simulink model "TorqueVect"  (R2022a)
settings: Solver=VariableStepAuto  StartTime=0.0  StopTime=32  RelTol=1e-3
PreLoadFcn:
  | run('Parameters\FSE_Parameters.m')
undefined symbols (not defined in the file): BRegenEnabledButton, canChannel, CyalphaLookUp, efficiency, Fz_curve, Fz_scaling_long, gearR, izz, jw, Kd, kd, Ki, ki, Kp, kp, l_f, l_r, lambda, m, Mz_max, N, N_lat, N_long, P_max, pid_kd_lat, pid_kd_long, pid_ki_lat, pid_ki_long, pid_kp_lat, pid_kp_long, R_max, rw, steerR, T_i_max, TC_Decr_Gas, TC_Derivative, TC_Incr_Gas, TC_On, TC_Relay_Off, TC_Relay_On, tireCornerStiffness, Ts, TV_On, TV_Override, velocity_lookup, velocity_lookup_lat, y_ref, yrr_scaling
libraries: simulink x218, slpidlib x135, CarMaker4SL x101, TractionControlLibrary x13, canmsglib x9, canlib x8, TorqueVectoringLibrary x6, simulink_extras x4, PedalConversionLibrary x3, PowerControlLibrary x1
(part 14 of 26)

== system TorqueVect/CarMaker/IPG Vehicle/PowerTrain/PTControl Example/PTControl_TV_MFE3/Full Control Loop/TC 4 ==
  modified slip ratio reference : Inport
  u_lim : Inport  Port=2
  modified slip ratio measurement : Inport  Port=3
  l_lim : Inport  Port=4
  ResetSignal : Inport  Port=5
  velocity : Inport  Port=6
  Constant : Constant  Value=kp
  Constant1 : Constant  Value=ki
  Constant2 : Constant  Value=kd
  Constant3 : Constant  Value=N
  PID Controller : slpidlib/PID Controller  Controller=PID  Form=Parallel  TimeDomain=Discrete-time  UseExternalTs=off  SampleTime=Ts  IntegratorMethod=Trapezoidal  FilterMethod=Forward Euler  ControllerParametersSource=external  P=kp  I=ki  UseKiTs=on  D=kd  N=100  UseFilter=on  TunerSelectOption=Transfer Function Based (PID Tuner App)  InitialConditionSource=internal  InitialConditionForIntegrator=0  InitialConditionForFilter=0  DifferentiatorICPrevScaledInput=0  ExternalReset=either  TrackingMode=off  Kt=1  LimitOutput=on  SatLimitsSource=external  UpperSaturationLimit=inf  LowerSaturationLimit=-inf  LinearizeAsGain=on  AntiWindupMode=clamping  Kb=1  POutMin=[]  POutMax=[]  IOutMin=[]  IOutMax=[]  DOutMin=[]  DOutMax=[]  NOutMin=[]  NOutMax=[]  SumOutMin=[]  SumOutMax=[]  SaturationOutMin=[]  SaturationOutMax=[]  PParamMin=[]  PParamMax=[]  IParamMin=[]  IParamMax=[]  DParamMin=[]  DParamMax=[]  NParamMin=[]  NParamMax=[]  KbParamMin=[]  KbParamMax=[]  KtParamMin=[]  KtParamMax=[]  KbOutMin=[]  KbOutMax=[]  KtOutMin=[]  KtOutMax=[]  IntegratorOutMin=[]  IntegratorOutMax=[]  FilterOutMin=[]  FilterOutMax=[]  SumI1OutMin=[]  SumI1OutMax=[]  SumI2OutMin=[]  SumI2OutMax=[]  SumI3OutMin=[]  SumI3OutMax=[]  SumI4OutMin=[]  SumI4OutMax=[]  SumDOutMin=[]  SumDOutMax=[]  DifferentiatorOutMin=[]  DifferentiatorOutMax=[]  FilterDiffOutCoefMin=[]  FilterDiffOutCoefMax=[]  ReciprocalOutMin=[]  ReciprocalOutMax=[]  SumDenOutMin=[]  SumDenOutMax=[]  SumNumOutMin=[]  SumNumOutMax=[]  DivideOutMin=[]  DivideOutMax=[]  UdiffTsProdOutMin=[]  UdiffTsProdOutMax=[]  NTsProdOutMin=[]  NTsProdOutMax=[]  UintegralTsProdOutMin=[]  UintegralTsProdOutMax=[]  UngainTsProdOutMin=[]  UngainTsProdOutMax=[]  ClampingZeroOutDataTypeStr=Inherit: Inherit via back propagation  ClampingZeroOutMin=[]  ClampingZeroOutMax=[]  FilterDenConstantOutDataTypeStr=Inherit: Inherit via back propagation  FilterDenConstantOutMin=[]  FilterDenConstantOutMax=[]  PCopyOutDataTypeStr=Inherit: Inherit via back propagation  PCopyOutMin=[]  PCopyOutMax=[]  NCopyOutDataTypeStr=Inherit: Inherit via back propagation  NCopyOutMin=[]  NCopyOutMax=[]  IntegratorContinuousStateAttributes=''  IntegratorStateMustResolveToSignalObject=off  IntegratorRTWStateStorageClass=Auto  FilterContinuousStateAttributes=''  FilterStateMustResolveToSignalObject=off  FilterRTWStateStorageClass=Auto  ParallelPVariant=ExternalParameters  IdealPVariant=Disabled  IVariant=ExternalParameters  DVariant=ExternalParameters  IntegratorVariant=Discrete  SatVariant=External  AWVariant=DiscClampingParallel  PCopyVariant=Disabled  TRVariant=Disabled  FdbkBlocksVariant=Feedback  IdealPFdbkVariant=Passthrough  SatFdbkVariant=Passthrough  DerivativeFilterVariant=ForwardEulerFilter  NVariant=ExternalParameters  NCopyVariant=Disabled  FilterICVariant=InternalICsFilter  IntegratorICVariant=InternalICs  ExternalResetVariant=ExternalReset  TRSumVariant=Passthrough  SumFdbkVariant=Enabled  SumVariant=Sum_PID  TsampFilterVariant=InternalTs  TsampNgainVariant=Passthrough  TsampIntegralVariant=Passthrough  ExternalSaturationOutDataTypeStr=Inherit: Same as second input  aMode=0
  Subsystem : Subsystem
  Sum1 : Sum  Inputs=|+-
  velocity lookup : Constant  Value=velocity_lookup
  Control Effort 1 : Outport
  wires:
  Sum1/1 -> PID Controller/1
  modified slip ratio reference/1 -> Sum1/1
  u_lim/1 -> PID Controller/7
  modified slip ratio measurement/1 -> Sum1/2
  l_lim/1 -> PID Controller/8
  PID Controller/1 -> Control Effort 1/1
  ResetSignal/1 -> PID Controller/6
  velocity/1 -> Subsystem/1(velocity)
  Constant/1 -> Subsystem/2(pid_kp)
  velocity lookup/1 -> Subsystem/3(velocity lookup)
  Subsystem/1(Out1) -> PID Controller/2
  Subsystem/2(Out2) -> PID Controller/3
  Subsystem/3(Out3) -> PID Controller/4
  Constant1/1 -> Subsystem/4(pid_ki)
  Constant2/1 -> Subsystem/5(pid_kd)
  Constant3/1 -> PID Controller/5

== system TorqueVect/CarMaker/IPG Vehicle/PowerTrain/PTControl Example/PTControl_TV_MFE3/New TC/Reference Generator1 ==
  note: For throttle sign and Product:
      | If positive, normal reference
      | If negative (regen), similar reference but negative (negative target slip*times speed), this might need to change to account for regen limits
      | If 0, target zero
  note: Vehicle velocity
  note: Modified slip ratio targets
  x2 : Inport
  Front SR Target : Inport  Port=2
  Rear SR Target : Inport  Port=3
  Constant : Constant
  Product1 : Product
  Product2 : Product
  Switch : Switch  Criteria=u2 > Threshold  Threshold=1  SaturateOnIntegerOverflow=off  InputSameDT=off
  R1 : Outport
  L1 : Outport  Port=2
  R2 : Outport  Port=3
  L2 : Outport  Port=4
  wires:
  Constant/1 -> Switch/3
  x2/1 -> Switch/2, Switch/1
  Switch/1 -> Product1/2, Product2/1
  Rear SR Target/1 -> Product2/2
  Product2/1 -> R2/1, L2/1
  Product1/1 -> R1/1, L1/1
  Front SR Target/1 -> Product1/1

== system TorqueVect/CarMaker/IPG Vehicle/PowerTrain/PTControl Example/PTControl_TV_MFE3/New TC/TC R1 ==
  modified slip ratio reference : Inport
  lim 1 : Inport  Port=2
  modified slip ratio measurement : Inport  Port=3
  P_TC : Inport  Port=4
  D_TC : Inport  Port=5
  enable_tc : Inport  Port=6
  PID Controller : slpidlib/PID Controller  Commented=on  Controller=PD  Form=Parallel  TimeDomain=Discrete-time  UseExternalTs=off  SampleTime=-1  IntegratorMethod=Forward Euler  FilterMethod=Forward Euler  ControllerParametersSource=external  P=125  I=1  UseKiTs=on  D=0  N=100  UseFilter=on  TunerSelectOption=Transfer Function Based (PID Tuner App)  InitialConditionSource=internal  InitialConditionForIntegrator=0  InitialConditionForFilter=0  DifferentiatorICPrevScaledInput=0  ExternalReset=none  TrackingMode=off  Kt=1  LimitOutput=on  SatLimitsSource=external  UpperSaturationLimit=inf  LowerSaturationLimit=-inf  LinearizeAsGain=on  AntiWindupMode=clamping  Kb=1  POutMin=[]  POutMax=[]  IOutMin=[]  IOutMax=[]  DOutMin=[]  DOutMax=[]  NOutMin=[]  NOutMax=[]  SumOutMin=[]  SumOutMax=[]  SaturationOutMin=[]  SaturationOutMax=[]  PParamMin=[]  PParamMax=[]  IParamMin=[]  IParamMax=[]  DParamMin=[]  DParamMax=[]  NParamMin=[]  NParamMax=[]  KbParamMin=[]  KbParamMax=[]  KtParamMin=[]  KtParamMax=[]  KbOutMin=[]  KbOutMax=[]  KtOutMin=[]  KtOutMax=[]  IntegratorOutMin=[]  IntegratorOutMax=[]  FilterOutMin=[]  FilterOutMax=[]  SumI1OutMin=[]  SumI1OutMax=[]  SumI2OutMin=[]  SumI2OutMax=[]  SumI3OutMin=[]  SumI3OutMax=[]  SumI4OutMin=[]  SumI4OutMax=[]  SumDOutMin=[]  SumDOutMax=[]  DifferentiatorOutMin=[]  DifferentiatorOutMax=[]  FilterDiffOutCoefMin=[]  FilterDiffOutCoefMax=[]  ReciprocalOutMin=[]  ReciprocalOutMax=[]  SumDenOutMin=[]  SumDenOutMax=[]  SumNumOutMin=[]  SumNumOutMax=[]  DivideOutMin=[]  DivideOutMax=[]  UdiffTsProdOutMin=[]  UdiffTsProdOutMax=[]  NTsProdOutMin=[]  NTsProdOutMax=[]  UintegralTsProdOutMin=[]  UintegralTsProdOutMax=[]  UngainTsProdOutMin=[]  UngainTsProdOutMax=[]  ClampingZeroOutDataTypeStr=Inherit: Inherit via back propagation  ClampingZeroOutMin=[]  ClampingZeroOutMax=[]  FilterDenConstantOutDataTypeStr=Inherit: Inherit via back propagation  FilterDenConstantOutMin=[]  FilterDenConstantOutMax=[]  PCopyOutDataTypeStr=Inherit: Inherit via back propagation  PCopyOutMin=[]  PCopyOutMax=[]  NCopyOutDataTypeStr=Inherit: Inherit via back propagation  NCopyOutMin=[]  NCopyOutMax=[]  IntegratorContinuousStateAttributes=''  IntegratorStateMustResolveToSignalObject=off  IntegratorRTWStateStorageClass=Auto  FilterContinuousStateAttributes=''  FilterStateMustResolveToSignalObject=off  FilterRTWStateStorageClass=Auto  ParallelPVariant=ExternalParameters  IdealPVariant=Disabled  IVariant=Disabled  DVariant=ExternalParameters  IntegratorVariant=Disabled  SatVariant=External  AWVariant=Disabled  PCopyVariant=Disabled  TRVariant=Disabled  FdbkBlocksVariant=Forward  IdealPFdbkVariant=Disabled  SatFdbkVariant=Disabled  DerivativeFilterVariant=ForwardEulerFilter  NVariant=ExternalParameters  NCopyVariant=Disabled  FilterICVariant=InternalICsFilter  IntegratorICVariant=Disabled  ExternalResetVariant=Disabled  TRSumVariant=Passthrough  SumFdbkVariant=Disabled  SumVariant=Sum_PD  TsampFilterVariant=InternalTs  TsampNgainVariant=Passthrough  TsampIntegralVariant=Disabled_SignalSpec  ExternalSaturationOutDataTypeStr=Inherit: Same as second input  aMode=0
  Sum1 : Sum  Inputs=|-+
  Sum2 : Sum  Commented=on  Inputs=|-+
  traction_controller : Subsystem
  Control Effort 1 : Outport
  wires:
  D_TC/1 -> traction_controller/5(Kd)
  P_TC/1 -> traction_controller/4(Kp)
  Sum1/1 -> traction_controller/2(dslip)
  enable_tc/1 -> traction_controller/3(enable_tc)
  traction_controller/1(delta_torque) -> Control Effort 1/1
  PID Controller/1 -> Sum2/1
  lim 1/1 -> traction_controller/1(max_torque), Sum2/2
  modified slip ratio measurement/1 -> Sum1/2
  modified slip ratio reference/1 -> Sum1/1

== system TorqueVect/CarMaker/IPG Vehicle/PowerTrain/PTControl Example/PTControl_TV_MFE3/New TC/TC R2 ==
  modified slip ratio reference : Inport
  lim 1 : Inport  Port=2
  modified slip ratio measurement : Inport  Port=3
  P_TC : Inport  Port=4
  D_TC : Inport  Port=5
  enable_tc : Inport  Port=6
  PID Controller : slpidlib/PID Controller  Commented=on  Controller=PD  Form=Parallel  TimeDomain=Discrete-time  UseExternalTs=off  SampleTime=-1  IntegratorMethod=Forward Euler  FilterMethod=Forward Euler  ControllerParametersSource=external  P=125  I=1  UseKiTs=on  D=0  N=100  UseFilter=on  TunerSelectOption=Transfer Function Based (PID Tuner App)  InitialConditionSource=internal  InitialConditionForIntegrator=0  InitialConditionForFilter=0  DifferentiatorICPrevScaledInput=0  ExternalReset=none  TrackingMode=off  Kt=1  LimitOutput=on  SatLimitsSource=external  UpperSaturationLimit=inf  LowerSaturationLimit=-inf  LinearizeAsGain=on  AntiWindupMode=clamping  Kb=1  POutMin=[]  POutMax=[]  IOutMin=[]  IOutMax=[]  DOutMin=[]  DOutMax=[]  NOutMin=[]  NOutMax=[]  SumOutMin=[]  SumOutMax=[]  SaturationOutMin=[]  SaturationOutMax=[]  PParamMin=[]  PParamMax=[]  IParamMin=[]  IParamMax=[]  DParamMin=[]  DParamMax=[]  NParamMin=[]  NParamMax=[]  KbParamMin=[]  KbParamMax=[]  KtParamMin=[]  KtParamMax=[]  KbOutMin=[]  KbOutMax=[]  KtOutMin=[]  KtOutMax=[]  IntegratorOutMin=[]  IntegratorOutMax=[]  FilterOutMin=[]  FilterOutMax=[]  SumI1OutMin=[]  SumI1OutMax=[]  SumI2OutMin=[]  SumI2OutMax=[]  SumI3OutMin=[]  SumI3OutMax=[]  SumI4OutMin=[]  SumI4OutMax=[]  SumDOutMin=[]  SumDOutMax=[]  DifferentiatorOutMin=[]  DifferentiatorOutMax=[]  FilterDiffOutCoefMin=[]  FilterDiffOutCoefMax=[]  ReciprocalOutMin=[]  ReciprocalOutMax=[]  SumDenOutMin=[]  SumDenOutMax=[]  SumNumOutMin=[]  SumNumOutMax=[]  DivideOutMin=[]  DivideOutMax=[]  UdiffTsProdOutMin=[]  UdiffTsProdOutMax=[]  NTsProdOutMin=[]  NTsProdOutMax=[]  UintegralTsProdOutMin=[]  UintegralTsProdOutMax=[]  UngainTsProdOutMin=[]  UngainTsProdOutMax=[]  ClampingZeroOutDataTypeStr=Inherit: Inherit via back propagation  ClampingZeroOutMin=[]  ClampingZeroOutMax=[]  FilterDenConstantOutDataTypeStr=Inherit: Inherit via back propagation  FilterDenConstantOutMin=[]  FilterDenConstantOutMax=[]  PCopyOutDataTypeStr=Inherit: Inherit via back propagation  PCopyOutMin=[]  PCopyOutMax=[]  NCopyOutDataTypeStr=Inherit: Inherit via back propagation  NCopyOutMin=[]  NCopyOutMax=[]  IntegratorContinuousStateAttributes=''  IntegratorStateMustResolveToSignalObject=off  IntegratorRTWStateStorageClass=Auto  FilterContinuousStateAttributes=''  FilterStateMustResolveToSignalObject=off  FilterRTWStateStorageClass=Auto  ParallelPVariant=ExternalParameters  IdealPVariant=Disabled  IVariant=Disabled  DVariant=ExternalParameters  IntegratorVariant=Disabled  SatVariant=External  AWVariant=Disabled  PCopyVariant=Disabled  TRVariant=Disabled  FdbkBlocksVariant=Forward  IdealPFdbkVariant=Disabled  SatFdbkVariant=Disabled  DerivativeFilterVariant=ForwardEulerFilter  NVariant=ExternalParameters  NCopyVariant=Disabled  FilterICVariant=InternalICsFilter  IntegratorICVariant=Disabled  ExternalResetVariant=Disabled  TRSumVariant=Passthrough  SumFdbkVariant=Disabled  SumVariant=Sum_PD  TsampFilterVariant=InternalTs  TsampNgainVariant=Passthrough  TsampIntegralVariant=Disabled_SignalSpec  ExternalSaturationOutDataTypeStr=Inherit: Same as second input  aMode=0
  Sum1 : Sum  Inputs=|-+
  Sum2 : Sum  Commented=on  Inputs=|-+
  traction_controller : Subsystem
  Control Effort 1 : Outport
  wires:
  D_TC/1 -> traction_controller/5(Kd)
  P_TC/1 -> traction_controller/4(Kp)
  Sum1/1 -> traction_controller/2(dslip)
  enable_tc/1 -> traction_controller/3(enable_tc)
  traction_controller/1(delta_torque) -> Control Effort 1/1
  PID Controller/1 -> Sum2/1
  lim 1/1 -> traction_controller/1(max_torque), Sum2/2
  modified slip ratio measurement/1 -> Sum1/2
  modified slip ratio reference/1 -> Sum1/1

== system TorqueVect/CarMaker/IPG Vehicle/PowerTrain/PTControl Example/PTControl_TV_MFE3/New TC/TC R3 ==
  modified slip ratio reference : Inport
  lim 1 : Inport  Port=2
  modified slip ratio measurement : Inport  Port=3
  P_TC : Inport  Port=4
  D_TC : Inport  Port=5
  enable_tc : Inport  Port=6
  PID Controller : slpidlib/PID Controller  Commented=on  Controller=PD  Form=Parallel  TimeDomain=Discrete-time  UseExternalTs=off  SampleTime=-1  IntegratorMethod=Forward Euler  FilterMethod=Forward Euler  ControllerParametersSource=external  P=125  I=1  UseKiTs=on  D=0  N=100  UseFilter=on  TunerSelectOption=Transfer Function Based (PID Tuner App)  InitialConditionSource=internal  InitialConditionForIntegrator=0  InitialConditionForFilter=0  DifferentiatorICPrevScaledInput=0  ExternalReset=none  TrackingMode=off  Kt=1  LimitOutput=on  SatLimitsSource=external  UpperSaturationLimit=inf  LowerSaturationLimit=-inf  LinearizeAsGain=on  AntiWindupMode=clamping  Kb=1  POutMin=[]  POutMax=[]  IOutMin=[]  IOutMax=[]  DOutMin=[]  DOutMax=[]  NOutMin=[]  NOutMax=[]  SumOutMin=[]  SumOutMax=[]  SaturationOutMin=[]  SaturationOutMax=[]  PParamMin=[]  PParamMax=[]  IParamMin=[]  IParamMax=[]  DParamMin=[]  DParamMax=[]  NParamMin=[]  NParamMax=[]  KbParamMin=[]  KbParamMax=[]  KtParamMin=[]  KtParamMax=[]  KbOutMin=[]  KbOutMax=[]  KtOutMin=[]  KtOutMax=[]  IntegratorOutMin=[]  IntegratorOutMax=[]  FilterOutMin=[]  FilterOutMax=[]  SumI1OutMin=[]  SumI1OutMax=[]  SumI2OutMin=[]  SumI2OutMax=[]  SumI3OutMin=[]  SumI3OutMax=[]  SumI4OutMin=[]  SumI4OutMax=[]  SumDOutMin=[]  SumDOutMax=[]  DifferentiatorOutMin=[]  DifferentiatorOutMax=[]  FilterDiffOutCoefMin=[]  FilterDiffOutCoefMax=[]  ReciprocalOutMin=[]  ReciprocalOutMax=[]  SumDenOutMin=[]  SumDenOutMax=[]  SumNumOutMin=[]  SumNumOutMax=[]  DivideOutMin=[]  DivideOutMax=[]  UdiffTsProdOutMin=[]  UdiffTsProdOutMax=[]  NTsProdOutMin=[]  NTsProdOutMax=[]  UintegralTsProdOutMin=[]  UintegralTsProdOutMax=[]  UngainTsProdOutMin=[]  UngainTsProdOutMax=[]  ClampingZeroOutDataTypeStr=Inherit: Inherit via back propagation  ClampingZeroOutMin=[]  ClampingZeroOutMax=[]  FilterDenConstantOutDataTypeStr=Inherit: Inherit via back propagation  FilterDenConstantOutMin=[]  FilterDenConstantOutMax=[]  PCopyOutDataTypeStr=Inherit: Inherit via back propagation  PCopyOutMin=[]  PCopyOutMax=[]  NCopyOutDataTypeStr=Inherit: Inherit via back propagation  NCopyOutMin=[]  NCopyOutMax=[]  IntegratorContinuousStateAttributes=''  IntegratorStateMustResolveToSignalObject=off  IntegratorRTWStateStorageClass=Auto  FilterContinuousStateAttributes=''  FilterStateMustResolveToSignalObject=off  FilterRTWStateStorageClass=Auto  ParallelPVariant=ExternalParameters  IdealPVariant=Disabled  IVariant=Disabled  DVariant=ExternalParameters  IntegratorVariant=Disabled  SatVariant=External  AWVariant=Disabled  PCopyVariant=Disabled  TRVariant=Disabled  FdbkBlocksVariant=Forward  IdealPFdbkVariant=Disabled  SatFdbkVariant=Disabled  DerivativeFilterVariant=ForwardEulerFilter  NVariant=ExternalParameters  NCopyVariant=Disabled  FilterICVariant=InternalICsFilter  IntegratorICVariant=Disabled  ExternalResetVariant=Disabled  TRSumVariant=Passthrough  SumFdbkVariant=Disabled  SumVariant=Sum_PD  TsampFilterVariant=InternalTs  TsampNgainVariant=Passthrough  TsampIntegralVariant=Disabled_SignalSpec  ExternalSaturationOutDataTypeStr=Inherit: Same as second input  aMode=0
  Sum1 : Sum  Inputs=|-+
  Sum2 : Sum  Commented=on  Inputs=|-+
  traction_controller : Subsystem
  Control Effort 1 : Outport
  wires:
  D_TC/1 -> traction_controller/5(Kd)
  P_TC/1 -> traction_controller/4(Kp)
  Sum1/1 -> traction_controller/2(dslip)
  enable_tc/1 -> traction_controller/3(enable_tc)
  traction_controller/1(delta_torque) -> Control Effort 1/1
  PID Controller/1 -> Sum2/1
  lim 1/1 -> traction_controller/1(max_torque), Sum2/2
  modified slip ratio measurement/1 -> Sum1/2
  modified slip ratio reference/1 -> Sum1/1

== system TorqueVect/CarMaker/IPG Vehicle/PowerTrain/PTControl Example/PTControl_TV_MFE3/New TC/TC R4 ==
  modified slip ratio reference : Inport
  lim 1 : Inport  Port=2
  modified slip ratio measurement : Inport  Port=3
  P_TC : Inport  Port=4
  D_TC : Inport  Port=5
  enable_tc : Inport  Port=6
  PID Controller : slpidlib/PID Controller  Commented=on  Controller=PD  Form=Parallel  TimeDomain=Discrete-time  UseExternalTs=off  SampleTime=-1  IntegratorMethod=Forward Euler  FilterMethod=Forward Euler  ControllerParametersSource=external  P=125  I=1  UseKiTs=on  D=0  N=100  UseFilter=on  TunerSelectOption=Transfer Function Based (PID Tuner App)  InitialConditionSource=internal  InitialConditionForIntegrator=0  InitialConditionForFilter=0  DifferentiatorICPrevScaledInput=0  ExternalReset=none  TrackingMode=off  Kt=1  LimitOutput=on  SatLimitsSource=external  UpperSaturationLimit=inf  LowerSaturationLimit=-inf  LinearizeAsGain=on  AntiWindupMode=clamping  Kb=1  POutMin=[]  POutMax=[]  IOutMin=[]  IOutMax=[]  DOutMin=[]  DOutMax=[]  NOutMin=[]  NOutMax=[]  SumOutMin=[]  SumOutMax=[]  SaturationOutMin=[]  SaturationOutMax=[]  PParamMin=[]  PParamMax=[]  IParamMin=[]  IParamMax=[]  DParamMin=[]  DParamMax=[]  NParamMin=[]  NParamMax=[]  KbParamMin=[]  KbParamMax=[]  KtParamMin=[]  KtParamMax=[]  KbOutMin=[]  KbOutMax=[]  KtOutMin=[]  KtOutMax=[]  IntegratorOutMin=[]  IntegratorOutMax=[]  FilterOutMin=[]  FilterOutMax=[]  SumI1OutMin=[]  SumI1OutMax=[]  SumI2OutMin=[]  SumI2OutMax=[]  SumI3OutMin=[]  SumI3OutMax=[]  SumI4OutMin=[]  SumI4OutMax=[]  SumDOutMin=[]  SumDOutMax=[]  DifferentiatorOutMin=[]  DifferentiatorOutMax=[]  FilterDiffOutCoefMin=[]  FilterDiffOutCoefMax=[]  ReciprocalOutMin=[]  ReciprocalOutMax=[]  SumDenOutMin=[]  SumDenOutMax=[]  SumNumOutMin=[]  SumNumOutMax=[]  DivideOutMin=[]  DivideOutMax=[]  UdiffTsProdOutMin=[]  UdiffTsProdOutMax=[]  NTsProdOutMin=[]  NTsProdOutMax=[]  UintegralTsProdOutMin=[]  UintegralTsProdOutMax=[]  UngainTsProdOutMin=[]  UngainTsProdOutMax=[]  ClampingZeroOutDataTypeStr=Inherit: Inherit via back propagation  ClampingZeroOutMin=[]  ClampingZeroOutMax=[]  FilterDenConstantOutDataTypeStr=Inherit: Inherit via back propagation  FilterDenConstantOutMin=[]  FilterDenConstantOutMax=[]  PCopyOutDataTypeStr=Inherit: Inherit via back propagation  PCopyOutMin=[]  PCopyOutMax=[]  NCopyOutDataTypeStr=Inherit: Inherit via back propagation  NCopyOutMin=[]  NCopyOutMax=[]  IntegratorContinuousStateAttributes=''  IntegratorStateMustResolveToSignalObject=off  IntegratorRTWStateStorageClass=Auto  FilterContinuousStateAttributes=''  FilterStateMustResolveToSignalObject=off  FilterRTWStateStorageClass=Auto  ParallelPVariant=ExternalParameters  IdealPVariant=Disabled  IVariant=Disabled  DVariant=ExternalParameters  IntegratorVariant=Disabled  SatVariant=External  AWVariant=Disabled  PCopyVariant=Disabled  TRVariant=Disabled  FdbkBlocksVariant=Forward  IdealPFdbkVariant=Disabled  SatFdbkVariant=Disabled  DerivativeFilterVariant=ForwardEulerFilter  NVariant=ExternalParameters  NCopyVariant=Disabled  FilterICVariant=InternalICsFilter  IntegratorICVariant=Disabled  ExternalResetVariant=Disabled  TRSumVariant=Passthrough  SumFdbkVariant=Disabled  SumVariant=Sum_PD  TsampFilterVariant=InternalTs  TsampNgainVariant=Passthrough  TsampIntegralVariant=Disabled_SignalSpec  ExternalSaturationOutDataTypeStr=Inherit: Same as second input  aMode=0
  Sum1 : Sum  Inputs=|-+
  Sum2 : Sum  Commented=on  Inputs=|-+
  traction_controller : Subsystem
  Control Effort 1 : Outport
  wires:
  D_TC/1 -> traction_controller/5(Kd)
  P_TC/1 -> traction_controller/4(Kp)
  Sum1/1 -> traction_controller/2(dslip)
  enable_tc/1 -> traction_controller/3(enable_tc)
  traction_controller/1(delta_torque) -> Control Effort 1/1
  PID Controller/1 -> Sum2/1
  lim 1/1 -> traction_controller/1(max_torque), Sum2/2
  modified slip ratio measurement/1 -> Sum1/2
  modified slip ratio reference/1 -> Sum1/1

== system TorqueVect/CarMaker/IPG Vehicle/PowerTrain/PTControl Example/PTControl_ALL_CTRL_VC_MFE24/New TC/TC R1/traction_controller ==
  max_torque : Inport
  dslip : Inport  Port=2
  enable_tc : Inport  Port=3
  Kp : Inport  Port=4
  Kd : Inport  Port=5
  Add : Sum  Inputs=+-
  Saturation Dynamic : simulink/Discontinuities/Saturation Dynamic  OutMin=[]  OutMax=[]  OutDataTypeStr=Inherit: Same as second input  OutDataType=fixdt(1, 16)  OutScaling=2^-10  DoSatur=off
  min_torque : Constant  Value=0
  traction_controller : Subsystem  TreatAsAtomicUnit=on
  delta_torque : Outport  VectorParamsAs1DForOutWhenUnconnected=off
  wires:
  Kd/1 -> traction_controller/4(Kd)
  enable_tc/1 -> traction_controller/2(enable_tc)
  Kp/1 -> traction_controller/3(Kp)
  traction_controller/1(delta_torque) -> Add/2
  dslip/1 -> traction_controller/1(dslip)
  Saturation Dynamic/1 -> delta_torque/1
  max_torque/1 -> Add/1, Saturation Dynamic/1
  min_torque/1 -> Saturation Dynamic/3
  Add/1 -> Saturation Dynamic/2

== system TorqueVect/CarMaker/IPG Vehicle/PowerTrain/PTControl Example/PTControl_ALL_CTRL_VC_MFE24/New TC/TC R2/traction_controller ==
  max_torque : Inport
  dslip : Inport  Port=2
  enable_tc : Inport  Port=3
  Kp : Inport  Port=4
  Kd : Inport  Port=5
  Add : Sum  Inputs=+-
  Saturation Dynamic : simulink/Discontinuities/Saturation Dynamic  OutMin=[]  OutMax=[]  OutDataTypeStr=Inherit: Same as second input  OutDataType=fixdt(1, 16)  OutScaling=2^-10  DoSatur=off
  min_torque : Constant  Value=0
  traction_controller : Subsystem  TreatAsAtomicUnit=on
  delta_torque : Outport  VectorParamsAs1DForOutWhenUnconnected=off
  wires:
  Kd/1 -> traction_controller/4(Kd)
  enable_tc/1 -> traction_controller/2(enable_tc)
  Kp/1 -> traction_controller/3(Kp)
  traction_controller/1(delta_torque) -> Add/2
  dslip/1 -> traction_controller/1(dslip)
  Saturation Dynamic/1 -> delta_torque/1
  max_torque/1 -> Add/1, Saturation Dynamic/1
  min_torque/1 -> Saturation Dynamic/3
  Add/1 -> Saturation Dynamic/2

== system TorqueVect/CarMaker/IPG Vehicle/PowerTrain/PTControl Example/PTControl_ALL_CTRL_VC_MFE24/New TC/TC R3/traction_controller ==
  max_torque : Inport
  dslip : Inport  Port=2
  enable_tc : Inport  Port=3
  Kp : Inport  Port=4
  Kd : Inport  Port=5
  Add : Sum  Inputs=+-
  Saturation Dynamic : simulink/Discontinuities/Saturation Dynamic  OutMin=[]  OutMax=[]  OutDataTypeStr=Inherit: Same as second input  OutDataType=fixdt(1, 16)  OutScaling=2^-10  DoSatur=off
  min_torque : Constant  Value=0
  traction_controller : Subsystem  TreatAsAtomicUnit=on
  delta_torque : Outport  VectorParamsAs1DForOutWhenUnconnected=off
  wires:
  Kd/1 -> traction_controller/4(Kd)
  enable_tc/1 -> traction_controller/2(enable_tc)
  Kp/1 -> traction_controller/3(Kp)
  traction_controller/1(delta_torque) -> Add/2
  dslip/1 -> traction_controller/1(dslip)
  Saturation Dynamic/1 -> delta_torque/1
  max_torque/1 -> Add/1, Saturation Dynamic/1
  min_torque/1 -> Saturation Dynamic/3
  Add/1 -> Saturation Dynamic/2

== system TorqueVect/CarMaker/IPG Vehicle/PowerTrain/PTControl Example/PTControl_ALL_CTRL_VC_MFE24/New TC/TC R4/traction_controller ==
  max_torque : Inport
  dslip : Inport  Port=2
  enable_tc : Inport  Port=3
  Kp : Inport  Port=4
  Kd : Inport  Port=5
  Add : Sum  Inputs=+-
  Saturation Dynamic : simulink/Discontinuities/Saturation Dynamic  OutMin=[]  OutMax=[]  OutDataTypeStr=Inherit: Same as second input  OutDataType=fixdt(1, 16)  OutScaling=2^-10  DoSatur=off
  min_torque : Constant  Value=0
  traction_controller : Subsystem  TreatAsAtomicUnit=on
  delta_torque : Outport  VectorParamsAs1DForOutWhenUnconnected=off
  wires:
  Kd/1 -> traction_controller/4(Kd)
  enable_tc/1 -> traction_controller/2(enable_tc)
  Kp/1 -> traction_controller/3(Kp)
  traction_controller/1(delta_torque) -> Add/2
  dslip/1 -> traction_controller/1(dslip)
  Saturation Dynamic/1 -> delta_torque/1
  max_torque/1 -> Add/1, Saturation Dynamic/1
  min_torque/1 -> Saturation Dynamic/3
  Add/1 -> Saturation Dynamic/2

== system TorqueVect/CarMaker/IPG Vehicle/PowerTrain/PTControl Example/PTControl_ALL_CTRL_VC_MFE24/Subsystem/PowerControl1/PC PID ==
  PError : Inport
  P_PC : Inport  Port=2
  D_PC : Inport  Port=3
  I_PC : Inport  Port=4
  ResetPID_PC : Inport  Port=5
  MMotorMax : Inport  Port=6
  Constant : Constant  Value=0
  Gain : Gain  Gain=4
  Gain1 : Gain  Gain=0.01
  PID Controller : slpidlib/PID Controller  Controller=PID  Form=Ideal  TimeDomain=Discrete-time  UseExternalTs=off  SampleTime=0.005  IntegratorMethod=Backward Euler  FilterMethod=Forward Euler  ControllerParametersSource=external  P=1  I=1  UseKiTs=on  D=0  N=100  UseFilter=off  TunerSelectOption=Transfer Function Based (PID Tuner App)  InitialConditionSource=internal  InitialConditionForIntegrator=0  InitialConditionForFilter=0  DifferentiatorICPrevScaledInput=0  ExternalReset=rising  TrackingMode=off  Kt=1  LimitOutput=on  SatLimitsSource=external  UpperSaturationLimit=84  LowerSaturationLimit=0  LinearizeAsGain=on  AntiWindupMode=clamping  Kb=2  SaturateOnIntegerOverflow=on  POutMin=[]  POutMax=[]  IOutMin=[]  IOutMax=[]  DOutMin=[]  DOutMax=[]  NOutMin=[]  NOutMax=[]  SumOutMin=[]  SumOutMax=[]  SaturationOutMin=[]  SaturationOutMax=[]  PParamMin=[]  PParamMax=[]  IParamMin=[]  IParamMax=[]  DParamMin=[]  DParamMax=[]  NParamMin=[]  NParamMax=[]  KbParamMin=[]  KbParamMax=[]  KtParamMin=[]  KtParamMax=[]  KbOutMin=[]  KbOutMax=[]  KtOutMin=[]  KtOutMax=[]  IntegratorOutMin=[]  IntegratorOutMax=[]  FilterOutMin=[]  FilterOutMax=[]  SumI1OutMin=[]  SumI1OutMax=[]  SumI2OutMin=[]  SumI2OutMax=[]  SumI3OutMin=[]  SumI3OutMax=[]  SumI4OutMin=[]  SumI4OutMax=[]  SumDOutMin=[]  SumDOutMax=[]  DifferentiatorOutMin=[]  DifferentiatorOutMax=[]  FilterDiffOutCoefMin=[]  FilterDiffOutCoefMax=[]  ReciprocalOutMin=[]  ReciprocalOutMax=[]  SumDenOutMin=[]  SumDenOutMax=[]  SumNumOutMin=[]  SumNumOutMax=[]  DivideOutMin=[]  DivideOutMax=[]  UdiffTsProdOutMin=[]  UdiffTsProdOutMax=[]  NTsProdOutMin=[]  NTsProdOutMax=[]  UintegralTsProdOutMin=[]  UintegralTsProdOutMax=[]  UngainTsProdOutMin=[]  UngainTsProdOutMax=[]  ClampingZeroOutDataTypeStr=Inherit: Inherit via back propagation  ClampingZeroOutMin=[]  ClampingZeroOutMax=[]  FilterDenConstantOutDataTypeStr=Inherit: Inherit via back propagation  FilterDenConstantOutMin=[]  FilterDenConstantOutMax=[]  PCopyOutDataTypeStr=Inherit: Inherit via back propagation  PCopyOutMin=[]  PCopyOutMax=[]  NCopyOutDataTypeStr=Inherit: Inherit via back propagation  NCopyOutMin=[]  NCopyOutMax=[]  IntegratorContinuousStateAttributes=''  IntegratorStateMustResolveToSignalObject=off  IntegratorRTWStateStorageClass=Auto  FilterContinuousStateAttributes=''  FilterStateMustResolveToSignalObject=off  FilterRTWStateStorageClass=Auto  ParallelPVariant=Passthrough  IdealPVariant=ExternalParameters  IVariant=ExternalParameters  DVariant=ExternalParameters  IntegratorVariant=Discrete  SatVariant=External  AWVariant=DiscClampingIdeal  PCopyVariant=ExternalParamsIdeal  TRVariant=Disabled  FdbkBlocksVariant=Feedback  IdealPFdbkVariant=ExternalParameters  SatFdbkVariant=Passthrough  DerivativeFilterVariant=Differentiator  NVariant=Passthrough  NCopyVariant=Disabled_SignalSpec  FilterICVariant=InternalICsDifferentiator  IntegratorICVariant=InternalICs  ExternalResetVariant=ExternalReset  TRSumVariant=Passthrough  SumFdbkVariant=Enabled  SumVariant=Sum_PID  TsampFilterVariant=InternalTs  TsampNgainVariant=Passthrough  TsampIntegralVariant=Passthrough  ExternalSaturationOutDataTypeStr=Inherit: Same as second input  aMode=0
  TrqReductionTotal : Outport
  wires:
  D_PC/1 -> PID Controller/4
  P_PC/1 -> PID Controller/2
  I_PC/1 -> PID Controller/3
  ResetPID_PC/1 -> PID Controller/5
  MMotorMax/1 -> Gain/1
  Gain/1 -> PID Controller/6
  Gain1/1 -> PID Controller/1
  PError/1 -> Gain1/1
  Constant/1 -> PID Controller/7
  PID Controller/1 -> TrqReductionTotal/1

== system TorqueVect/CarMaker/IPG Vehicle/PowerTrain/PTControl Example/PTControl_ALL_CTRL_VC_MFE24/Subsystem/PowerControl1/PID1 ==
  PError : Inport
  PRegenError : Inport  Port=2
  P_PC : Inport  Port=3
  D_PC : Inport  Port=4
  I_PC : Inport  Port=5
  ResetPID_PC : Inport  Port=6
  MMotorMax : Inport  Port=7
  BRegenEnabled : Inport  Port=8
  rThrottlePedal : Inport  Port=9
  AND : Logic  IconShape=distinctive  AllPortsSameDT=off  OutDataTypeStr=boolean
  Add : Sum
  Compare To Constant : simulink/Logic and Bit Operations/Compare To Constant  relop=<=  const=0.1  OutDataTypeStr=boolean
  Constant : Constant  Value=0
  Gain : Gain  Gain=4
  Gain1 : Gain  Gain=0.01
  Gain2 : Gain  Gain=-1
  PID Controller : slpidlib/PID Controller  Controller=PID  Form=Ideal  TimeDomain=Discrete-time  UseExternalTs=off  SampleTime=0.005  IntegratorMethod=Backward Euler  FilterMethod=Forward Euler  ControllerParametersSource=external  P=1  I=1  UseKiTs=on  D=0  N=100  UseFilter=off  TunerSelectOption=Transfer Function Based (PID Tuner App)  InitialConditionSource=internal  InitialConditionForIntegrator=0  InitialConditionForFilter=0  DifferentiatorICPrevScaledInput=0  ExternalReset=rising  TrackingMode=off  Kt=1  LimitOutput=on  SatLimitsSource=external  UpperSaturationLimit=84  LowerSaturationLimit=0  LinearizeAsGain=on  AntiWindupMode=clamping  Kb=2  SaturateOnIntegerOverflow=on  POutMin=[]  POutMax=[]  IOutMin=[]  IOutMax=[]  DOutMin=[]  DOutMax=[]  NOutMin=[]  NOutMax=[]  SumOutMin=[]  SumOutMax=[]  SaturationOutMin=[]  SaturationOutMax=[]  PParamMin=[]  PParamMax=[]  IParamMin=[]  IParamMax=[]  DParamMin=[]  DParamMax=[]  NParamMin=[]  NParamMax=[]  KbParamMin=[]  KbParamMax=[]  KtParamMin=[]  KtParamMax=[]  KbOutMin=[]  KbOutMax=[]  KtOutMin=[]  KtOutMax=[]  IntegratorOutMin=[]  IntegratorOutMax=[]  FilterOutMin=[]  FilterOutMax=[]  SumI1OutMin=[]  SumI1OutMax=[]  SumI2OutMin=[]  SumI2OutMax=[]  SumI3OutMin=[]  SumI3OutMax=[]  SumI4OutMin=[]  SumI4OutMax=[]  SumDOutMin=[]  SumDOutMax=[]  DifferentiatorOutMin=[]  DifferentiatorOutMax=[]  FilterDiffOutCoefMin=[]  FilterDiffOutCoefMax=[]  ReciprocalOutMin=[]  ReciprocalOutMax=[]  SumDenOutMin=[]  SumDenOutMax=[]  SumNumOutMin=[]  SumNumOutMax=[]  DivideOutMin=[]  DivideOutMax=[]  UdiffTsProdOutMin=[]  UdiffTsProdOutMax=[]  NTsProdOutMin=[]  NTsProdOutMax=[]  UintegralTsProdOutMin=[]  UintegralTsProdOutMax=[]  UngainTsProdOutMin=[]  UngainTsProdOutMax=[]  ClampingZeroOutDataTypeStr=Inherit: Inherit via back propagation  ClampingZeroOutMin=[]  ClampingZeroOutMax=[]  FilterDenConstantOutDataTypeStr=Inherit: Inherit via back propagation  FilterDenConstantOutMin=[]  FilterDenConstantOutMax=[]  PCopyOutDataTypeStr=Inherit: Inherit via back propagation  PCopyOutMin=[]  PCopyOutMax=[]  NCopyOutDataTypeStr=Inherit: Inherit via back propagation  NCopyOutMin=[]  NCopyOutMax=[]  IntegratorContinuousStateAttributes=''  IntegratorStateMustResolveToSignalObject=off  IntegratorRTWStateStorageClass=Auto  FilterContinuousStateAttributes=''  FilterStateMustResolveToSignalObject=off  FilterRTWStateStorageClass=Auto  ParallelPVariant=Passthrough  IdealPVariant=ExternalParameters  IVariant=ExternalParameters  DVariant=ExternalParameters  IntegratorVariant=Discrete  SatVariant=External  AWVariant=DiscClampingIdeal  PCopyVariant=ExternalParamsIdeal  TRVariant=Disabled  FdbkBlocksVariant=Feedback  IdealPFdbkVariant=ExternalParameters  SatFdbkVariant=Passthrough  DerivativeFilterVariant=Differentiator  NVariant=Passthrough  NCopyVariant=Disabled_SignalSpec  FilterICVariant=InternalICsDifferentiator  IntegratorICVariant=InternalICs  ExternalResetVariant=ExternalReset  TRSumVariant=Passthrough  SumFdbkVariant=Enabled  SumVariant=Sum_PID  TsampFilterVariant=InternalTs  TsampNgainVariant=Passthrough  TsampIntegralVariant=Passthrough  ExternalSaturationOutDataTypeStr=Inherit: Same as second input  aMode=0
  Switch : Switch  Criteria=u2 > Threshold  SaturateOnIntegerOverflow=off  InputSameDT=off
  TrqReductionTotal : Outport
  wires:
  ? -> TrqReductionTotal/1  "control input delta_P"
  D_PC/1 -> ?
  P_PC/1 -> ?
  I_PC/1 -> ?
  ResetPID_PC/1 -> ?
  MMotorMax/1 -> Gain/1
  Gain/1 -> Gain2/1
  Gain1/1 -> ?
  Add/1 -> Gain1/1
  PError/1 -> Add/1
  PRegenError/1 -> Add/2
  rThrottlePedal/1 -> ?
  BRegenEnabled/1 -> AND/1
  ? -> AND/2
  AND/1 -> Switch/2
  Switch/1 -> ?
  Constant/1 -> Switch/3
  Gain2/1 -> Switch/1

== system TorqueVect/CarMaker/IPG Vehicle/PowerTrain/PTControl Example/PTControl_ALL_CTRL_VC_MFE24/Subsystem/PowerControl1/PowerError ==
  PPositiveTotal : Inport  Unit=W  PortDimensions=1
      settings: AttributesFormatString=%<Unit>
  FF_PC : Inport  Port=2
  PLimit : Inport  Port=3  OutMin=0  OutMax=80000  Unit=W  PortDimensions=1
      settings: AttributesFormatString=[%<OutMin>, %<OutMax>] %<Unit>
  Product5 : Product
  Saturation2 : Saturate  UpperLimit=250000  LowerLimit=0
      settings: AttributesFormatString=[%<LowerLimit>, %<UpperLimit>] W
  Subtract2 : Sum  Inputs=+-
  PError : Outport  Unit=W  PortDimensions=1
      settings: AttributesFormatString=%<Unit>
  wires:
  FF_PC/1 -> Product5/2
  Subtract2/1 -> Saturation2/1
  PLimit/1 -> Subtract2/2
  PPositiveTotal/1 -> Product5/1
  Saturation2/1 -> PError/1  "power error"
  Product5/1 -> Subtract2/1

== system TorqueVect/CarMaker/IPG Vehicle/PowerTrain/PTControl Example/PTControl_ALL_CTRL_VC_MFE24/Subsystem/PowerControl1/RC PID ==
  PRegenError : Inport
  P_RC : Inport  Port=2
  D_RC : Inport  Port=3
  I_RC : Inport  Port=4
  ResetPID_RC : Inport  Port=5
  MRegenMotorMax : Inport  Port=6
  Constant : Constant  Value=0
  Gain : Gain  Gain=-4
  Gain1 : Gain  Gain=-0.01
  PID Controller : slpidlib/PID Controller  Controller=PID  Form=Ideal  TimeDomain=Discrete-time  UseExternalTs=off  SampleTime=0.005  IntegratorMethod=Backward Euler  FilterMethod=Forward Euler  ControllerParametersSource=external  P=1  I=1  UseKiTs=on  D=0  N=100  UseFilter=off  TunerSelectOption=Transfer Function Based (PID Tuner App)  InitialConditionSource=internal  InitialConditionForIntegrator=0  InitialConditionForFilter=0  DifferentiatorICPrevScaledInput=0  ExternalReset=level  TrackingMode=off  Kt=1  LimitOutput=on  SatLimitsSource=external  UpperSaturationLimit=84  LowerSaturationLimit=0  LinearizeAsGain=on  AntiWindupMode=clamping  Kb=2  SaturateOnIntegerOverflow=on  POutMin=[]  POutMax=[]  IOutMin=[]  IOutMax=[]  DOutMin=[]  DOutMax=[]  NOutMin=[]  NOutMax=[]  SumOutMin=[]  SumOutMax=[]  SaturationOutMin=[]  SaturationOutMax=[]  PParamMin=[]  PParamMax=[]  IParamMin=[]  IParamMax=[]  DParamMin=[]  DParamMax=[]  NParamMin=[]  NParamMax=[]  KbParamMin=[]  KbParamMax=[]  KtParamMin=[]  KtParamMax=[]  KbOutMin=[]  KbOutMax=[]  KtOutMin=[]  KtOutMax=[]  IntegratorOutMin=[]  IntegratorOutMax=[]  FilterOutMin=[]  FilterOutMax=[]  SumI1OutMin=[]  SumI1OutMax=[]  SumI2OutMin=[]  SumI2OutMax=[]  SumI3OutMin=[]  SumI3OutMax=[]  SumI4OutMin=[]  SumI4OutMax=[]  SumDOutMin=[]  SumDOutMax=[]  DifferentiatorOutMin=[]  DifferentiatorOutMax=[]  FilterDiffOutCoefMin=[]  FilterDiffOutCoefMax=[]  ReciprocalOutMin=[]  ReciprocalOutMax=[]  SumDenOutMin=[]  SumDenOutMax=[]  SumNumOutMin=[]  SumNumOutMax=[]  DivideOutMin=[]  DivideOutMax=[]  UdiffTsProdOutMin=[]  UdiffTsProdOutMax=[]  NTsProdOutMin=[]  NTsProdOutMax=[]  UintegralTsProdOutMin=[]  UintegralTsProdOutMax=[]  UngainTsProdOutMin=[]  UngainTsProdOutMax=[]  ClampingZeroOutDataTypeStr=Inherit: Inherit via back propagation  ClampingZeroOutMin=[]  ClampingZeroOutMax=[]  FilterDenConstantOutDataTypeStr=Inherit: Inherit via back propagation  FilterDenConstantOutMin=[]  FilterDenConstantOutMax=[]  PCopyOutDataTypeStr=Inherit: Inherit via back propagation  PCopyOutMin=[]  PCopyOutMax=[]  NCopyOutDataTypeStr=Inherit: Inherit via back propagation  NCopyOutMin=[]  NCopyOutMax=[]  IntegratorContinuousStateAttributes=''  IntegratorStateMustResolveToSignalObject=off  IntegratorRTWStateStorageClass=Auto  FilterContinuousStateAttributes=''  FilterStateMustResolveToSignalObject=off  FilterRTWStateStorageClass=Auto  ParallelPVariant=Passthrough  IdealPVariant=ExternalParameters  IVariant=ExternalParameters  DVariant=ExternalParameters  IntegratorVariant=Discrete  SatVariant=External  AWVariant=DiscClampingIdeal  PCopyVariant=ExternalParamsIdeal  TRVariant=Disabled  FdbkBlocksVariant=Feedback  IdealPFdbkVariant=ExternalParameters  SatFdbkVariant=Passthrough  DerivativeFilterVariant=Differentiator  NVariant=Passthrough  NCopyVariant=Disabled_SignalSpec  FilterICVariant=InternalICsDifferentiator  IntegratorICVariant=InternalICs  ExternalResetVariant=ExternalReset  TRSumVariant=Passthrough  SumFdbkVariant=Enabled  SumVariant=Sum_PID  TsampFilterVariant=InternalTs  TsampNgainVariant=Passthrough  TsampIntegralVariant=Passthrough  ExternalSaturationOutDataTypeStr=Inherit: Same as second input  aMode=0
  RegenTrqReductionTotal : Outport
  wires:
  D_RC/1 -> PID Controller/4
  P_RC/1 -> PID Controller/2
  I_RC/1 -> PID Controller/3
  ResetPID_RC/1 -> PID Controller/5
  Gain1/1 -> PID Controller/1
  PRegenError/1 -> Gain1/1
  MRegenMotorMax/1 -> Gain/1
  Constant/1 -> PID Controller/6
  Gain/1 -> PID Controller/7
  PID Controller/1 -> RegenTrqReductionTotal/1

== system TorqueVect/CarMaker/IPG Vehicle/PowerTrain/PTControl Example/PTControl_ALL_CTRL_VC_MFE24/Subsystem/PowerControl1/RegenError ==
  PTotal : Inport  Unit=W  PortDimensions=1
      settings: AttributesFormatString=%<Unit>
  FF_RC : Inport  Port=2
  PRegenLimit : Inport  Port=3  OutMin=0  OutMax=80000  Unit=W  PortDimensions=1
      settings: AttributesFormatString=[%<OutMin>, %<OutMax>] %<Unit>
  rThrottle : Inport  Port=4
  BRegenEnable : Inport  Port=5
  Product : Product
  Product1 : Product
  Product6 : Product
  Saturation : Saturate  UpperLimit=0  LowerLimit=-250000
  Saturation7 : Saturate  UpperLimit=0  LowerLimit=-250000
      settings: AttributesFormatString=[%<LowerLimit>, %<UpperLimit>] W
  Subtract1 : Sum  Inputs=+-
  PRegenError : Outport  Unit=W  PortDimensions=1
      settings: AttributesFormatString=%<Unit>
  wires:
  Saturation/1 -> Subtract1/2
  PRegenLimit/1 -> Product/2
  rThrottle/1 -> Product/1
  Product/1 -> Saturation/1
  Subtract1/1 -> Saturation7/1
  PTotal/1 -> Product6/1
  Product6/1 -> Subtract1/1
  FF_RC/1 -> Product6/2
  Product1/1 -> PRegenError/1
  Saturation7/1 -> Product1/1  "regen error"
  BRegenEnable/1 -> Product1/2

== system TorqueVect/CarMaker/IPG Vehicle/PowerTrain/PTControl Example/PTControl_ALL_CTRL_VC_MFE24/Subsystem/PowerControl1/ResetPID_PC ==
  note: Resets when the pedal is below pos torque demand and there is still a reduction by the PID
  note: Resets when the pedal is in the idle zone [8-11%]
  rThrottlePedal : Inport
  PReductionTotal : Inport  Port=2
  AND : Logic  IconShape=distinctive  AllPortsSameDT=off  OutDataTypeStr=boolean
  AND1 : Logic  Inputs=3  IconShape=distinctive  AllPortsSameDT=off  OutDataTypeStr=boolean
  Compare To Constant1 : simulink/Logic and Bit Operations/Compare To Constant  relop=<=  const=0.1  OutDataTypeStr=boolean
  Compare To Constant2 : simulink/Logic and Bit Operations/Compare To Constant  relop=<=  const=0.11  OutDataTypeStr=boolean
  Compare To Constant3 : simulink/Logic and Bit Operations/Compare To Constant  relop=>=  const=0.08  OutDataTypeStr=boolean
  Compare To Constant4 : simulink/Logic and Bit Operations/Compare To Constant  relop=>  const=0  OutDataTypeStr=boolean
  Detect Fall Negative1 : simulink/Logic and Bit Operations/Detect Fall Negative  vinit=0  OutDataTypeStr=boolean
      settings: SourceProductBaseCode=SL
  Discrete Derivative1 : simulink/Discrete/Discrete Derivative  gainval=1.0  ICPrevScaledInput=0.0  OutMin=[]  OutMax=[]  OutDataType=fixdt(1, 16)  OutScaling=2^-10  DoSatur=off
  OR : Logic  Operator=OR  IconShape=distinctive  AllPortsSameDT=off  OutDataTypeStr=boolean
  ResetPID_PC : Outport
  wires:
  rThrottlePedal/1 -> Compare To Constant2/1, Discrete Derivative1/1, Compare To Constant3/1, Compare To Constant1/1
  OR/1 -> ResetPID_PC/1
  PReductionTotal/1 -> Compare To Constant4/1
  AND1/1 -> OR/1
  AND/1 -> OR/2
  Compare To Constant2/1 -> AND1/3
  Discrete Derivative1/1 -> Detect Fall Negative1/1
  Detect Fall Negative1/1 -> AND1/2
  Compare To Constant3/1 -> AND/1
  Compare To Constant1/1 -> AND/2

== system TorqueVect/CarMaker/IPG Vehicle/PowerTrain/PTControl Example/PTControl_ALL_CTRL_VC_MFE24/Subsystem/PowerControl1/ResetPID_RC ==
  note: Resets when the pedal is above regen torque demand and there is still a reaction by the PID
  note: Resets when regen becomes disabled
  note: Resets when the pedal is in the idle zone [8-11%]
  rThrottlePedal1 : Inport
  RegenTrqReductionTotal1 : Inport  Port=2
  BRegenEnabled1 : Inport  Port=3
  Current : Inport  Port=4
  AND2 : Logic  IconShape=distinctive  AllPortsSameDT=off  OutDataTypeStr=boolean
  AND3 : Logic  Inputs=3  IconShape=distinctive  AllPortsSameDT=off  OutDataTypeStr=boolean
  Compare To Constant10 : simulink/Logic and Bit Operations/Compare To Constant  relop=<  const=0  OutDataTypeStr=boolean
  Compare To Constant11 : simulink/Logic and Bit Operations/Compare To Constant  relop=>=  const=0  OutDataTypeStr=boolean
  Compare To Constant6 : simulink/Logic and Bit Operations/Compare To Constant  relop===  const=0  OutDataTypeStr=boolean
  Compare To Constant7 : simulink/Logic and Bit Operations/Compare To Constant  relop=>=  const=0.07  OutDataTypeStr=boolean
  Compare To Constant8 : simulink/Logic and Bit Operations/Compare To Constant  relop=<=  const=0.1  OutDataTypeStr=boolean
  Compare To Constant9 : simulink/Logic and Bit Operations/Compare To Constant  relop=>=  const=0.07  OutDataTypeStr=boolean
  Detect Fall Negative1 : simulink/Logic and Bit Operations/Detect Fall Negative  vinit=0  OutDataTypeStr=boolean
      settings: SourceProductBaseCode=SL
  Detect Rise Positive1 : simulink/Logic and Bit Operations/Detect Rise Positive  vinit=0  OutDataTypeStr=boolean
  Discrete Derivative2 : simulink/Discrete/Discrete Derivative  gainval=1.0  ICPrevScaledInput=0.0  OutMin=[]  OutMax=[]  OutDataType=fixdt(1, 16)  OutScaling=2^-10  DoSatur=off
  OR2 : Logic  Operator=OR  Inputs=4  IconShape=distinctive  AllPortsSameDT=off  OutDataTypeStr=boolean
  OR3 : Logic  Operator=OR  IconShape=distinctive  AllPortsSameDT=off  OutDataTypeStr=boolean
  ResetPID_RC1 : Outport
  wires:
  AND3/1 -> OR2/2
  BRegenEnabled1/1 -> Compare To Constant6/1, Detect Fall Negative1/1
  Compare To Constant7/1 -> AND2/1
  Compare To Constant9/1 -> AND3/3
  Detect Fall Negative1/1 -> OR3/2
  Compare To Constant6/1 -> OR3/1
  Current/1 -> Compare To Constant11/1
  Compare To Constant11/1 -> OR2/4
  Detect Rise Positive1/1 -> AND3/2  "accel_pedal_rising_or"
  OR2/1 -> ResetPID_RC1/1
  OR3/1 -> OR2/1
  AND2/1 -> OR2/3
  Compare To Constant8/1 -> AND3/1
  Discrete Derivative2/1 -> Detect Rise Positive1/1
  RegenTrqReductionTotal1/1 -> Compare To Constant10/1
  Compare To Constant10/1 -> AND2/2
  rThrottlePedal1/1 -> Compare To Constant7/1, Compare To Constant9/1, Compare To Constant8/1, Discrete Derivative2/1

== system TorqueVect/CarMaker/IPG Vehicle/PowerTrain/PTControl Example/PTControl_ALL_CTRL_VC_MFE24/Subsystem/PowerControl1/Subsystem ==
  TrqReductionTotal : Inport
  rSplitF : Inport  Port=2
  Constant : Constant
  Product : Product
  Sum : Sum  Inputs=|+-
  Sum1 : Sum  Inputs=|-+
  TrqReductionR : Outport
  TrqReductionF : Outport  Port=2
  wires:
  TrqReductionTotal/1 -> Product/1, Sum/1
  Product/1 -> TrqReductionF/1, Sum/2
  Sum/1 -> TrqReductionR/1
  rSplitF/1 -> Sum1/1
  Constant/1 -> Sum1/2
  Sum1/1 -> Product/2

== system TorqueVect/CarMaker/IPG Vehicle/PowerTrain/PTControl Example/PTControl_ALL_CTRL_VC_MFE24/Subsystem/PowerControl1/TotalPower ==
  PMeasured : Inport  OutMin=-250000  OutMax=250000  Unit=W  PortDimensions=1
      settings: AttributesFormatString=[%<OutMin>, %<OutMax>] %<Unit>
  Saturation5 : Saturate  UpperLimit=250000  LowerLimit=0
  PPositiveTotal : Outport  OutMin=0  OutMax=250000  Unit=W  PortDimensions=1
      settings: AttributesFormatString=[%<OutMin>, %<OutMax>] %<Unit>
  PTotal : Outport  Port=2
  wires:
  PMeasured/1 -> PTotal/1, Saturation5/1
  Saturation5/1 -> PPositiveTotal/1

== system TorqueVect/CarMaker/IPG Vehicle/PowerTrain/PTControl Example/PTControl_ALL_CTRL_VC_MFE24/Subsystem/PowerControl2/PC PID ==
  PError : Inport
  P_PC : Inport  Port=2
  D_PC : Inport  Port=3
  I_PC : Inport  Port=4
  ResetPID_PC : Inport  Port=5
  MMotorMax : Inport  Port=6
  Constant : Constant  Value=0
  Gain : Gain  Gain=4
  Gain1 : Gain  Gain=0.01
  PID Controller : slpidlib/PID Controller  Controller=PID  Form=Ideal  TimeDomain=Discrete-time  UseExternalTs=off  SampleTime=0.005  IntegratorMethod=Backward Euler  FilterMethod=Forward Euler  ControllerParametersSource=external  P=1  I=1  UseKiTs=on  D=0  N=100  UseFilter=off  TunerSelectOption=Transfer Function Based (PID Tuner App)  InitialConditionSource=internal  InitialConditionForIntegrator=0  InitialConditionForFilter=0  DifferentiatorICPrevScaledInput=0  ExternalReset=rising  TrackingMode=off  Kt=1  LimitOutput=on  SatLimitsSource=external  UpperSaturationLimit=84  LowerSaturationLimit=0  LinearizeAsGain=on  AntiWindupMode=clamping  Kb=2  SaturateOnIntegerOverflow=on  POutMin=[]  POutMax=[]  IOutMin=[]  IOutMax=[]  DOutMin=[]  DOutMax=[]  NOutMin=[]  NOutMax=[]  SumOutMin=[]  SumOutMax=[]  SaturationOutMin=[]  SaturationOutMax=[]  PParamMin=[]  PParamMax=[]  IParamMin=[]  IParamMax=[]  DParamMin=[]  DParamMax=[]  NParamMin=[]  NParamMax=[]  KbParamMin=[]  KbParamMax=[]  KtParamMin=[]  KtParamMax=[]  KbOutMin=[]  KbOutMax=[]  KtOutMin=[]  KtOutMax=[]  IntegratorOutMin=[]  IntegratorOutMax=[]  FilterOutMin=[]  FilterOutMax=[]  SumI1OutMin=[]  SumI1OutMax=[]  SumI2OutMin=[]  SumI2OutMax=[]  SumI3OutMin=[]  SumI3OutMax=[]  SumI4OutMin=[]  SumI4OutMax=[]  SumDOutMin=[]  SumDOutMax=[]  DifferentiatorOutMin=[]  DifferentiatorOutMax=[]  FilterDiffOutCoefMin=[]  FilterDiffOutCoefMax=[]  ReciprocalOutMin=[]  ReciprocalOutMax=[]  SumDenOutMin=[]  SumDenOutMax=[]  SumNumOutMin=[]  SumNumOutMax=[]  DivideOutMin=[]  DivideOutMax=[]  UdiffTsProdOutMin=[]  UdiffTsProdOutMax=[]  NTsProdOutMin=[]  NTsProdOutMax=[]  UintegralTsProdOutMin=[]  UintegralTsProdOutMax=[]  UngainTsProdOutMin=[]  UngainTsProdOutMax=[]  ClampingZeroOutDataTypeStr=Inherit: Inherit via back propagation  ClampingZeroOutMin=[]  ClampingZeroOutMax=[]  FilterDenConstantOutDataTypeStr=Inherit: Inherit via back propagation  FilterDenConstantOutMin=[]  FilterDenConstantOutMax=[]  PCopyOutDataTypeStr=Inherit: Inherit via back propagation  PCopyOutMin=[]  PCopyOutMax=[]  NCopyOutDataTypeStr=Inherit: Inherit via back propagation  NCopyOutMin=[]  NCopyOutMax=[]  IntegratorContinuousStateAttributes=''  IntegratorStateMustResolveToSignalObject=off  IntegratorRTWStateStorageClass=Auto  FilterContinuousStateAttributes=''  FilterStateMustResolveToSignalObject=off  FilterRTWStateStorageClass=Auto  ParallelPVariant=Passthrough  IdealPVariant=ExternalParameters  IVariant=ExternalParameters  DVariant=ExternalParameters  IntegratorVariant=Discrete  SatVariant=External  AWVariant=DiscClampingIdeal  PCopyVariant=ExternalParamsIdeal  TRVariant=Disabled  FdbkBlocksVariant=Feedback  IdealPFdbkVariant=ExternalParameters  SatFdbkVariant=Passthrough  DerivativeFilterVariant=Differentiator  NVariant=Passthrough  NCopyVariant=Disabled_SignalSpec  FilterICVariant=InternalICsDifferentiator  IntegratorICVariant=InternalICs  ExternalResetVariant=ExternalReset  TRSumVariant=Passthrough  SumFdbkVariant=Enabled  SumVariant=Sum_PID  TsampFilterVariant=InternalTs  TsampNgainVariant=Passthrough  TsampIntegralVariant=Passthrough  ExternalSaturationOutDataTypeStr=Inherit: Same as second input  aMode=0
  TrqReductionTotal : Outport
  wires:
  ? -> TrqReductionTotal/1  "control input delta_P"
  D_PC/1 -> ?
  P_PC/1 -> ?
  I_PC/1 -> ?
  ResetPID_PC/1 -> ?
  MMotorMax/1 -> Gain/1
  Gain/1 -> ?
  Gain1/1 -> ?
  PError/1 -> Gain1/1
  Constant/1 -> ?
